simulink model "simulation"  (R2023b)
settings: Solver=VariableStepAuto  StartTime=0.0  StopTime=10.0  RelTol=1e-3
libraries: eeLuenbergerObserver x1
settings Model: Creator=adama  LastModifiedBy=adama

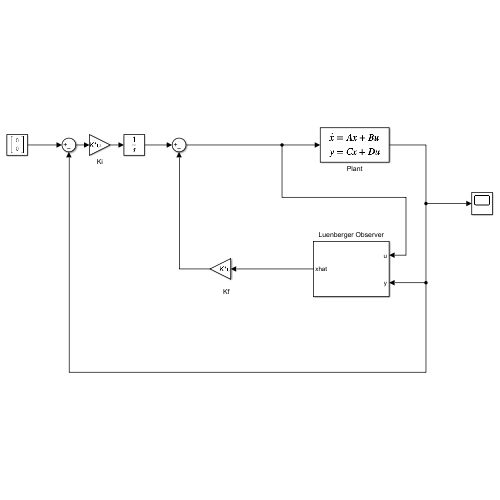
[thumbnail: Simulink's stored preview of the top-level diagram]
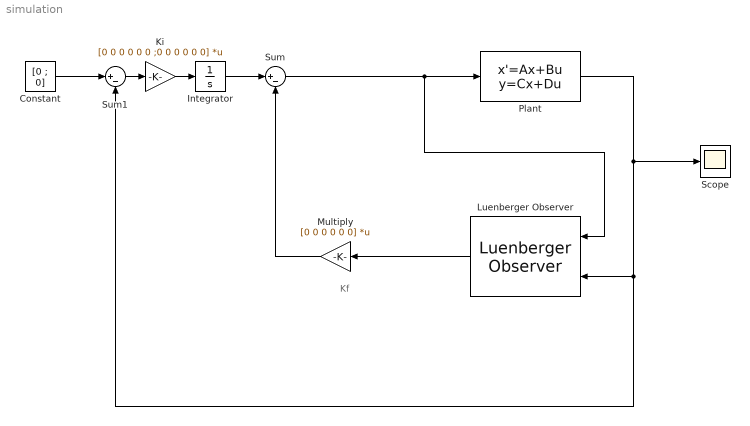
== system simulation ==
  note: Kf
  Constant : Constant  Value=[0 ; 0]  VectorParams1D=off
  Integrator : Integrator
  Ki : Gain  Gain=[0 0 0 0 0 0 ;0 0 0 0 0 0]  Multiplication=Matrix(K*u)
  Luenberger Observer : eeLuenbergerObserver/Luenberger Observer  StateSpaceType=Discrete-time  Ad=1  Bd=1  Cd=1  Dd=1  A=1  B=1  C=1  D=1  ObserverDesign=Desired eigenvalues  Ld=1  DesiredEigenvalues=0  x0=0  Tsd=0.1  Ts=0.1
      settings: LibrarySourceBlock=ee_sl_lib/Observers/Luenberger Observer
  Multiply : Gain  Gain=[0 0 0 0 0 0]  Multiplication=Matrix(K*u)
  Plant : StateSpace  InitialCondition=0
  Scope : Scope
  Sum : Sum  Inputs=|+-
  Sum1 : Sum  Inputs=|+-
  wires:
  Luenberger Observer/1 -> Multiply/1
  Plant/1 -> Scope/1, Luenberger Observer/2, Sum1/2
  Multiply/1 -> Sum/2
  Sum/1 -> Luenberger Observer/1, Plant/1
  Sum1/1 -> Ki/1
  Constant/1 -> Sum1/1
  Ki/1 -> Integrator/1
  Integrator/1 -> Sum/1
